simulink model "cruise_control_PIDmodel"  (R2020a)
settings: Solver=ode15s  StartTime=0.0  StopTime=10.0  RelTol=1e-3
values from neighbouring files (symbols this model uses):
  b = 50    [workspace_data.mat]
  kd = 1    [workspace_data.mat]
  ki = 40    [workspace_data.mat]
  kp = 800    [workspace_data.mat]
  m = 1000    [workspace_data.mat]
settings Model: Creator=shweta  LastModifiedBy=shweta

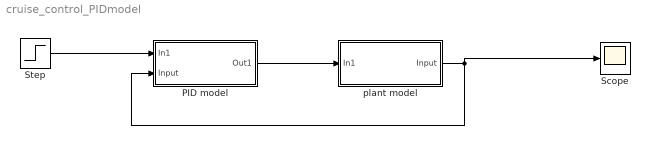
== system cruise_control_PIDmodel ==
  PID model : Subsystem  TreatAsAtomicUnit=on
  Scope : Scope
  Step : Step  Time=0
  plant model : Subsystem
  wires:
  Step/1 -> PID model/1(In1)
  plant model/1(Input) -> Scope/1, PID model/2(Input)
  PID model/1(Out1) -> plant model/1(In1)

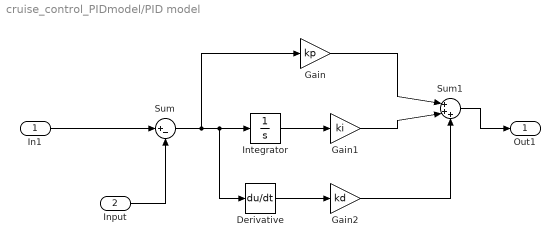
== system cruise_control_PIDmodel/PID model ==
  In1 : Inport  SampleTime=0
  Input : Inport  Port=2
  Derivative : Derivative
  Gain : Gain  Gain=kp
  Gain1 : Gain  Gain=ki
  Gain2 : Gain  Gain=kd
  Integrator : Integrator
  Sum : Sum  Inputs=|+-
  Sum1 : Sum  Inputs=|+++
  Out1 : Outport
  wires:
  Sum/1 -> Gain/1, Derivative/1, Integrator/1
  Input/1 -> Sum/2
  Gain1/1 -> Sum1/2
  Integrator/1 -> Gain1/1
  Sum1/1 -> Out1/1
  Gain/1 -> Sum1/1
  In1/1 -> Sum/1
  Derivative/1 -> Gain2/1
  Gain2/1 -> Sum1/3

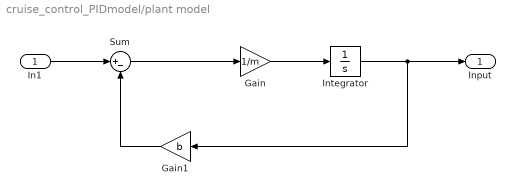
== system cruise_control_PIDmodel/plant model ==
  In1 : Inport
  Gain : Gain  Gain=1/m
  Gain1 : Gain  Gain=b
  Integrator : Integrator
  Sum : Sum  Inputs=|+-
  Input : Outport
  wires:
  In1/1 -> Sum/1
  Gain1/1 -> Sum/2
  Sum/1 -> Gain/1
  Gain/1 -> Integrator/1
  Integrator/1 -> Gain1/1, Input/1
